simulink model "active_with_narx_and_can"  (R2024a)
settings: Solver=FixedStepAuto  StartTime=0.0  StopTime=40  FixedStep=0.005  RelTol=1e-3
undefined symbols (not defined in the file): A, B, C, canChannel, D, E, H, K1, K2, params, VehicleDataSingle
libraries: neural x41, j1939protocollib x5, vntj1939tllib x1, sldrtlib x1, simulink x1
(part 3 of 3)

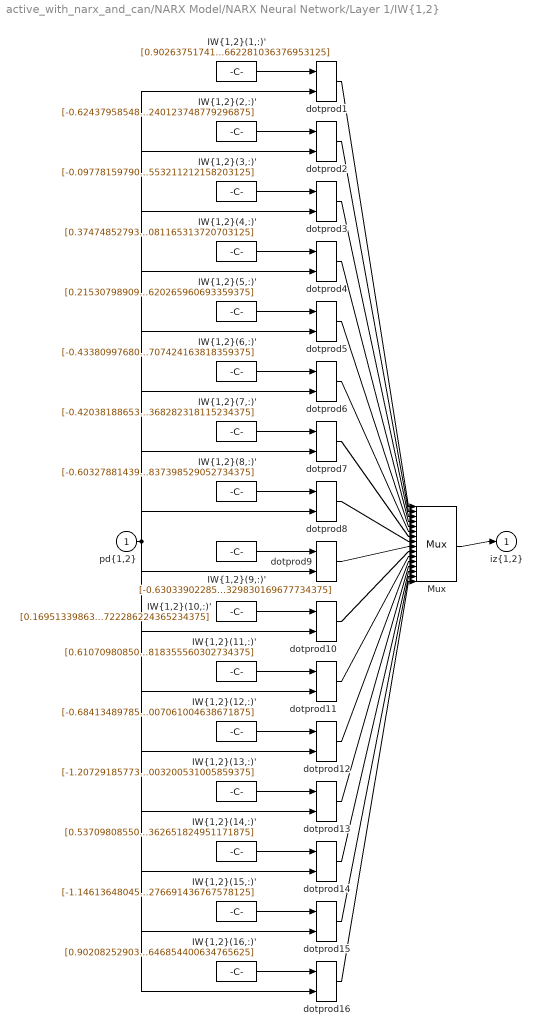
== system active_with_narx_and_can/NARX Model/NARX Neural Network/Layer 1/IW{1,2} ==
  "pd{1,2}" : Inport  PortDimensions=8
      mask Display: e = 0.06;c1 = [120 230 180]/255;c2 = ([120 230 180]+0)/(256+128);c3 = ([120 230 180]+128)/(256+128);patch([0 1 1 0],[0 0 1 1],c1);patch([0 1 1 1-e 1-e 0+e],[0 0 1 1-e 0+e 0+e],c2);patch([0 0 1 1-e 0+e 0+e],[0 1 1 1-e 1-e 0+e],c3);plot([0 1 1 0 0],[0 0 1 1 0]);
  "IW{1,2}(1,:)'" : Constant  Value=[0.90263751741286313290402176789939403533935546875;-0.21601499662720013983374656163505278527736663818359375;0.303445752325211037803143199198530055582523345947265625;-0.485376444032000919914793257703422568738460540771484375;0.23563832005407914227390619998914189636707305908203125;0.2294133098908705259422191602425300516188144683837890625;0.25051304698929321990163998634670861065387725830078125;0.1704435947606100232309955799792078323662281036376953125]
      mask Display: e = 0.06;c1 = [120 150 230]/255;c2 = ([120 150 230]+0)/383;c3 = ([120 150 230]+128)/383;patch([0 1 1 0],[0 0 1 1],c1);patch([0 1 1 1-e 1-e 0+e],[0 0 1 1-e 0+e 0+e],c2);patch([0 0 1 1-e 0+e 0+e],[0 1 1 1-e 1-e 0+e],c3);plot([0 1 1 0 0],[0 0 1 1 0]);disp('Weights');
  "IW{1,2}(10,:)'" : Constant  Value=[0.169513398630651845877537198248319327831268310546875;-1.0365359109949310312259740385343320667743682861328125;0.11236096590994171240396326538757421076297760009765625;-0.55860279468901430366400973070994950830936431884765625;0.40321310435647372827361323288641870021820068359375;0.2438622089058629927027510575499036349356174468994140625;0.218310799669648336607252758767572231590747833251953125;0.1471962379093022244003208243157132528722286224365234375]
      mask Display: e = 0.06;c1 = [120 150 230]/255;c2 = ([120 150 230]+0)/383;c3 = ([120 150 230]+128)/383;patch([0 1 1 0],[0 0 1 1],c1);patch([0 1 1 1-e 1-e 0+e],[0 0 1 1-e 0+e 0+e],c2);patch([0 0 1 1-e 0+e 0+e],[0 1 1 1-e 1-e 0+e],c3);plot([0 1 1 0 0],[0 0 1 1 0]);disp('Weights');
  "IW{1,2}(11,:)'" : Constant  Value=[0.61070980850982314880326384809450246393680572509765625;-0.6571629666322793550392589168041013181209564208984375;-0.292207907782760123449605771384085528552532196044921875;-0.6071086591404124543913667366723529994487762451171875;-0.7255795782161500451223901109187863767147064208984375;-0.10046686132956735015842042457734351046383380889892578125;-0.29501543782765649037713728830567561089992523193359375;-0.057419468308792909194693265817477367818355560302734375]
      mask Display: e = 0.06;c1 = [120 150 230]/255;c2 = ([120 150 230]+0)/383;c3 = ([120 150 230]+128)/383;patch([0 1 1 0],[0 0 1 1],c1);patch([0 1 1 1-e 1-e 0+e],[0 0 1 1-e 0+e 0+e],c2);patch([0 0 1 1-e 0+e 0+e],[0 1 1 1-e 1-e 0+e],c3);plot([0 1 1 0 0],[0 0 1 1 0]);disp('Weights');
  "IW{1,2}(12,:)'" : Constant  Value=[-0.68413489785069703241759953016298823058605194091796875;0.7251253878621028992057517825742252171039581298828125;-0.2162451686483140844696748672504327259957790374755859375;1.14689883587164676015390796237625181674957275390625;1.4145020007900115377452721077133901417255401611328125;-0.269077578797319028058865342245553620159626007080078125;0.00336010815578813813730985060601597069762647151947021484375;0.18742002039583638417497013506363146007061004638671875]
      mask Display: e = 0.06;c1 = [120 150 230]/255;c2 = ([120 150 230]+0)/383;c3 = ([120 150 230]+128)/383;patch([0 1 1 0],[0 0 1 1],c1);patch([0 1 1 1-e 1-e 0+e],[0 0 1 1-e 0+e 0+e],c2);patch([0 0 1 1-e 0+e 0+e],[0 1 1 1-e 1-e 0+e],c3);plot([0 1 1 0 0],[0 0 1 1 0]);disp('Weights');
  "IW{1,2}(13,:)'" : Constant  Value=[-1.207291857736213724905383060104213654994964599609375;-0.01499466201103569380770341723518868093378841876983642578125;-0.173091376080131309489473778739920817315578460693359375;0.282268142750107420280158976311213336884975433349609375;1.1083543211750790380420994551968760788440704345703125;-0.00180324813542519723184864854914621901116333901882171630859375;-0.4755764174158214618870488266111351549625396728515625;-0.696182258878252469003200531005859375]
      mask Display: e = 0.06;c1 = [120 150 230]/255;c2 = ([120 150 230]+0)/383;c3 = ([120 150 230]+128)/383;patch([0 1 1 0],[0 0 1 1],c1);patch([0 1 1 1-e 1-e 0+e],[0 0 1 1-e 0+e 0+e],c2);patch([0 0 1 1-e 0+e 0+e],[0 1 1 1-e 1-e 0+e],c3);plot([0 1 1 0 0],[0 0 1 1 0]);disp('Weights');
  "IW{1,2}(14,:)'" : Constant  Value=[0.5370980855067768455768373314640484750270843505859375;-0.313056847114534908538274748934782110154628753662109375;0.0770138039934813445341887927497737109661102294921875;0.64018782705027021950883181489189155399799346923828125;-0.07635916492874746108743266859164577908813953399658203125;0.0942864795317774895266893508960492908954620361328125;-0.09106729824357506775101001039729453623294830322265625;0.42317469894027837096217581347445957362651824951171875]
      mask Display: e = 0.06;c1 = [120 150 230]/255;c2 = ([120 150 230]+0)/383;c3 = ([120 150 230]+128)/383;patch([0 1 1 0],[0 0 1 1],c1);patch([0 1 1 1-e 1-e 0+e],[0 0 1 1-e 0+e 0+e],c2);patch([0 0 1 1-e 0+e 0+e],[0 1 1 1-e 1-e 0+e],c3);plot([0 1 1 0 0],[0 0 1 1 0]);disp('Weights');
  "IW{1,2}(15,:)'" : Constant  Value=[-1.146136480454412076568360134842805564403533935546875;-0.0944942787904399228438023783382959663867950439453125;-0.3428836995163557777033247475628741085529327392578125;-0.7923366916232279510978742109728045761585235595703125;-0.06468206728460264287594583265672554261982440948486328125;0.60584543936818746612260611072997562587261199951171875;0.768091475662020517489736448624171316623687744140625;0.63206824404375716586201860991423018276691436767578125]
      mask Display: e = 0.06;c1 = [120 150 230]/255;c2 = ([120 150 230]+0)/383;c3 = ([120 150 230]+128)/383;patch([0 1 1 0],[0 0 1 1],c1);patch([0 1 1 1-e 1-e 0+e],[0 0 1 1-e 0+e 0+e],c2);patch([0 0 1 1-e 0+e 0+e],[0 1 1 1-e 1-e 0+e],c3);plot([0 1 1 0 0],[0 0 1 1 0]);disp('Weights');
  "IW{1,2}(16,:)'" : Constant  Value=[0.90208252903466756844608198662172071635723114013671875;-0.36075579545011626780848246198729611933231353759765625;-0.47607267246013462713705166606814600527286529541015625;-0.4239340155265429732622806113795377314090728759765625;0.323166192061411561287087579330545850098133087158203125;-0.417318695834025199520311844025854952633380889892578125;-0.79057600537506467208714866501395590603351593017578125;-0.72856943152513642392165138517157174646854400634765625]
      mask Display: e = 0.06;c1 = [120 150 230]/255;c2 = ([120 150 230]+0)/383;c3 = ([120 150 230]+128)/383;patch([0 1 1 0],[0 0 1 1],c1);patch([0 1 1 1-e 1-e 0+e],[0 0 1 1-e 0+e 0+e],c2);patch([0 0 1 1-e 0+e 0+e],[0 1 1 1-e 1-e 0+e],c3);plot([0 1 1 0 0],[0 0 1 1 0]);disp('Weights');
  "IW{1,2}(2,:)'" : Constant  Value=[-0.62437958548816696602301590246497653424739837646484375;0.4030010330402535867477809006231836974620819091796875;-0.93345120950187820962895557386218570172786712646484375;-0.99941077496806574043120008354890160262584686279296875;-0.805871382932370039497982361353933811187744140625;-1.1641510599605722209304303760291077196598052978515625;-0.73810501632568803476175389732816256582736968994140625;-0.52273946016513750389975712096202187240123748779296875]
      mask Display: e = 0.06;c1 = [120 150 230]/255;c2 = ([120 150 230]+0)/383;c3 = ([120 150 230]+128)/383;patch([0 1 1 0],[0 0 1 1],c1);patch([0 1 1 1-e 1-e 0+e],[0 0 1 1-e 0+e 0+e],c2);patch([0 0 1 1-e 0+e 0+e],[0 1 1 1-e 1-e 0+e],c3);plot([0 1 1 0 0],[0 0 1 1 0]);disp('Weights');
  "IW{1,2}(3,:)'" : Constant  Value=[-0.09778159790864258960052524116690619848668575286865234375;-0.385707484802180811112037872590008191764354705810546875;0.7925023952755034795103483702405355870723724365234375;0.51074010904656663711875808076001703739166259765625;-0.68969065456008837866619387568789534270763397216796875;-0.00582392983700102083444161138459094217978417873382568359375;0.1302174028268628103166548726221662946045398712158203125;0.1331059726587587033197479513546568341553211212158203125]
      mask Display: e = 0.06;c1 = [120 150 230]/255;c2 = ([120 150 230]+0)/383;c3 = ([120 150 230]+128)/383;patch([0 1 1 0],[0 0 1 1],c1);patch([0 1 1 1-e 1-e 0+e],[0 0 1 1-e 0+e 0+e],c2);patch([0 0 1 1-e 0+e 0+e],[0 1 1 1-e 1-e 0+e],c3);plot([0 1 1 0 0],[0 0 1 1 0]);disp('Weights');
  "IW{1,2}(4,:)'" : Constant  Value=[0.37474852793019242103156329903868027031421661376953125;0.2591676118072852030849162474623881280422210693359375;-0.2053060696935578022248591878451406955718994140625;0.2190438597914983187564530453528277575969696044921875;-0.06545895398947572385583981713352841325104236602783203125;-0.2064269491545067669591162484721280634403228759765625;-0.11894725401665766362224729846275295130908489227294921875;0.0374038305425073158705373543853056617081165313720703125]
      mask Display: e = 0.06;c1 = [120 150 230]/255;c2 = ([120 150 230]+0)/383;c3 = ([120 150 230]+128)/383;patch([0 1 1 0],[0 0 1 1],c1);patch([0 1 1 1-e 1-e 0+e],[0 0 1 1-e 0+e 0+e],c2);patch([0 0 1 1-e 0+e 0+e],[0 1 1 1-e 1-e 0+e],c3);plot([0 1 1 0 0],[0 0 1 1 0]);disp('Weights');
  "IW{1,2}(5,:)'" : Constant  Value=[0.21530798909694393028502190645667724311351776123046875;-0.896805076954492630392223873059265315532684326171875;0.433263582933134439034716933747404254972934722900390625;-0.180462695486016289070363427526899613440036773681640625;0.32220381062158953699992025576648302376270294189453125;-0.1843317232416837592179348348508938215672969818115234375;0.35367194604087914822088123401044867932796478271484375;0.42561556904118302835371423498145304620265960693359375]
      mask Display: e = 0.06;c1 = [120 150 230]/255;c2 = ([120 150 230]+0)/383;c3 = ([120 150 230]+128)/383;patch([0 1 1 0],[0 0 1 1],c1);patch([0 1 1 1-e 1-e 0+e],[0 0 1 1-e 0+e 0+e],c2);patch([0 0 1 1-e 0+e 0+e],[0 1 1 1-e 1-e 0+e],c3);plot([0 1 1 0 0],[0 0 1 1 0]);disp('Weights');
  "IW{1,2}(6,:)'" : Constant  Value=[-0.433809976807434882761782546367612667381763458251953125;-0.270578592932165740148064969616825692355632781982421875;-0.4396279200653336882709254496148787438869476318359375;0.0907362057473349026270881267919321544468402862548828125;0.251838525357704512419587672411580570042133331298828125;-0.02289131637670037411336210197987384162843227386474609375;0.1623517875336642768413497606161399744451045989990234375;0.08045006984227652535590635807238868437707424163818359375]
      mask Display: e = 0.06;c1 = [120 150 230]/255;c2 = ([120 150 230]+0)/383;c3 = ([120 150 230]+128)/383;patch([0 1 1 0],[0 0 1 1],c1);patch([0 1 1 1-e 1-e 0+e],[0 0 1 1-e 0+e 0+e],c2);patch([0 0 1 1-e 0+e 0+e],[0 1 1 1-e 1-e 0+e],c3);plot([0 1 1 0 0],[0 0 1 1 0]);disp('Weights');
  "IW{1,2}(7,:)'" : Constant  Value=[-0.420381886532580295590122432258795015513896942138671875;0.18477735142202422746748879944789223372936248779296875;-0.48409542286411000322488007441279478371143341064453125;-0.2112447543197915333923475600386154837906360626220703125;-0.1131105735586611371612519860718748532235622406005859375;-0.268798366024736612445167338592000305652618408203125;-0.136020135754542526029808868770487606525421142578125;-0.0886993300823918084940800099502666853368282318115234375]
      mask Display: e = 0.06;c1 = [120 150 230]/255;c2 = ([120 150 230]+0)/383;c3 = ([120 150 230]+128)/383;patch([0 1 1 0],[0 0 1 1],c1);patch([0 1 1 1-e 1-e 0+e],[0 0 1 1-e 0+e 0+e],c2);patch([0 0 1 1-e 0+e 0+e],[0 1 1 1-e 1-e 0+e],c3);plot([0 1 1 0 0],[0 0 1 1 0]);disp('Weights');
  "IW{1,2}(8,:)'" : Constant  Value=[-0.603278814390159734415419734432362020015716552734375;0.1260379163613980224578625666254083625972270965576171875;0.227830739133030368837040668950066901743412017822265625;0.72188803288705416516535251503228209912776947021484375;0.942978873146900209434306816547177731990814208984375;0.9617318813040556246818368890671990811824798583984375;-0.386824720566464275162132935292902402579784393310546875;-0.0515663129788129503960902866310789249837398529052734375]
      mask Display: e = 0.06;c1 = [120 150 230]/255;c2 = ([120 150 230]+0)/383;c3 = ([120 150 230]+128)/383;patch([0 1 1 0],[0 0 1 1],c1);patch([0 1 1 1-e 1-e 0+e],[0 0 1 1-e 0+e 0+e],c2);patch([0 0 1 1-e 0+e 0+e],[0 1 1 1-e 1-e 0+e],c3);plot([0 1 1 0 0],[0 0 1 1 0]);disp('Weights');
  "IW{1,2}(9,:)'" : Constant  Value=[-0.63033902285547060984072231804020702838897705078125;-0.5593934237156599209583873744122684001922607421875;-0.413146987113548858072675784569582901895046234130859375;0.14086159676361831305513305778731591999530792236328125;-0.612650184316847035148612121702171862125396728515625;1.1652010827542447213289733554120175540447235107421875;-0.667181620491609894685325343743897974491119384765625;-0.51448630339249967757808690294041298329830169677734375]
      mask Display: e = 0.06;c1 = [120 150 230]/255;c2 = ([120 150 230]+0)/383;c3 = ([120 150 230]+128)/383;patch([0 1 1 0],[0 0 1 1],c1);patch([0 1 1 1-e 1-e 0+e],[0 0 1 1-e 0+e 0+e],c2);patch([0 0 1 1-e 0+e 0+e],[0 1 1 1-e 1-e 0+e],c3);plot([0 1 1 0 0],[0 0 1 1 0]);disp('Weights');
  Mux : Mux  Inputs=16
      mask Display: e = 0.06;c1 = [120 150 230]/255;c2 = ([120 150 230]+0)/383;c3 = ([120 150 230]+128)/383;patch([0 1 1 0],[0 0 1 1],c1);patch([0 1 1 1-e 1-e 0+e],[0 0 1 1-e 0+e 0+e],c2);patch([0 0 1 1-e 0+e 0+e],[0 1 1 1-e 1-e 0+e],c3);plot([0 1 1 0 0],[0 0 1 1 0]);disp('Mux');
  dotprod{1..16} (16 alike) : neural/Weight Functions/dotprod
  "iz{1,2}" : Outport
      mask Display: e = 0.06;c1 = [120 230 180]/255;c2 = ([120 230 180]+0)/(256+128);c3 = ([120 230 180]+128)/(256+128);patch([0 1 1 0],[0 0 1 1],c1);patch([0 1 1 1-e 1-e 0+e],[0 0 1 1-e 0+e 0+e],c2);patch([0 0 1 1-e 0+e 0+e],[0 1 1 1-e 1-e 0+e],c3);plot([0 1 1 0 0],[0 0 1 1 0]);
  wires:
  "IW{1,2}(1,:)'"/1 -> dotprod1/1
  "pd{1,2}"/1 -> dotprod1/2, dotprod2/2, dotprod3/2, dotprod4/2, dotprod5/2, dotprod6/2, dotprod7/2, dotprod8/2, dotprod9/2, dotprod10/2, dotprod11/2, dotprod12/2, dotprod13/2, dotprod14/2, dotprod15/2, dotprod16/2
  dotprod1/1 -> Mux/1
  "IW{1,2}(2,:)'"/1 -> dotprod2/1
  dotprod2/1 -> Mux/2
  "IW{1,2}(3,:)'"/1 -> dotprod3/1
  dotprod3/1 -> Mux/3
  "IW{1,2}(4,:)'"/1 -> dotprod4/1
  dotprod4/1 -> Mux/4
  "IW{1,2}(5,:)'"/1 -> dotprod5/1
  dotprod5/1 -> Mux/5
  "IW{1,2}(6,:)'"/1 -> dotprod6/1
  dotprod6/1 -> Mux/6
  "IW{1,2}(7,:)'"/1 -> dotprod7/1
  dotprod7/1 -> Mux/7
  "IW{1,2}(8,:)'"/1 -> dotprod8/1
  dotprod8/1 -> Mux/8
  "IW{1,2}(9,:)'"/1 -> dotprod9/1
  dotprod9/1 -> Mux/9
  "IW{1,2}(10,:)'"/1 -> dotprod10/1
  dotprod10/1 -> Mux/10
  "IW{1,2}(11,:)'"/1 -> dotprod11/1
  dotprod11/1 -> Mux/11
  "IW{1,2}(12,:)'"/1 -> dotprod12/1
  dotprod12/1 -> Mux/12
  "IW{1,2}(13,:)'"/1 -> dotprod13/1
  dotprod13/1 -> Mux/13
  "IW{1,2}(14,:)'"/1 -> dotprod14/1
  dotprod14/1 -> Mux/14
  "IW{1,2}(15,:)'"/1 -> dotprod15/1
  dotprod15/1 -> Mux/15
  "IW{1,2}(16,:)'"/1 -> dotprod16/1
  dotprod16/1 -> Mux/16
  Mux/1 -> "iz{1,2}"/1

== system active_with_narx_and_can/NARX Model/NARX Neural Network/Layer 2/Delays 1 ==
  "p{2}" : Inport  PortDimensions=16
      mask Display: e = 0.06;c1 = [120 230 180]/255;c2 = ([120 230 180]+0)/(256+128);c3 = ([120 230 180]+128)/(256+128);patch([0 1 1 0],[0 0 1 1],c1);patch([0 1 1 1-e 1-e 0+e],[0 0 1 1-e 0+e 0+e],c2);patch([0 0 1 1-e 0+e 0+e],[0 1 1 1-e 1-e 0+e],c3);plot([0 1 1 0 0],[0 0 1 1 0]);
  mux : Mux  Inputs=1
      mask Display: e = 0.06;c1 = [120 150 230]/255;c2 = ([120 150 230]+0)/383;c3 = ([120 150 230]+128)/383;patch([0 1 1 0],[0 0 1 1],c1);patch([0 1 1 1-e 1-e 0+e],[0 0 1 1-e 0+e 0+e],c2);patch([0 0 1 1-e 0+e 0+e],[0 1 1 1-e 1-e 0+e],c3);plot([0 1 1 0 0],[0 0 1 1 0]);disp('Mux')
  "pd{2,1}" : Outport
      mask Display: e = 0.06;c1 = [120 230 180]/255;c2 = ([120 230 180]+0)/(256+128);c3 = ([120 230 180]+128)/(256+128);patch([0 1 1 0],[0 0 1 1],c1);patch([0 1 1 1-e 1-e 0+e],[0 0 1 1-e 0+e 0+e],c2);patch([0 0 1 1-e 0+e 0+e],[0 1 1 1-e 1-e 0+e],c3);plot([0 1 1 0 0],[0 0 1 1 0]);
  wires:
  "p{2}"/1 -> mux/1
  mux/1 -> "pd{2,1}"/1

== system active_with_narx_and_can/NARX Model/NARX Neural Network/Layer 2/LW{2,1} ==
  "ad{2,1}" : Inport  PortDimensions=16
      mask Display: e = 0.06;c1 = [120 230 180]/255;c2 = ([120 230 180]+0)/(256+128);c3 = ([120 230 180]+128)/(256+128);patch([0 1 1 0],[0 0 1 1],c1);patch([0 1 1 1-e 1-e 0+e],[0 0 1 1-e 0+e 0+e],c2);patch([0 0 1 1-e 0+e 0+e],[0 1 1 1-e 1-e 0+e],c3);plot([0 1 1 0 0],[0 0 1 1 0]);
  "IW{2,1}(1,:)'" : Constant  Value=[-0.037283359326283883883323966301759355701506137847900390625;-0.00752528952071175420701631963993349927477538585662841796875;-0.064064462501762398094484751709387637674808502197265625;1.062458244357101566635037670494057238101959228515625;0.035078437349624867758191015809643431566655635833740234375;-0.0231289547996484136371808659760063164867460727691650390625;-0.86705623148364552310596309325774200260639190673828125;-0.1254112477086657129188296266875113360583782196044921875;0.041761451141637866146805180278533953242003917694091796875;-0.159013841309073866714385303566814400255680084228515625;0.15100937644207623744563306900090537965297698974609375;-0.08639823493543609400635574502302915789186954498291015625;0.381990846404795636459539309726096689701080322265625;0.041620895665299674492931814029361703433096408843994140625;0.69392710050268091581671114909113384783267974853515625;0.32302310650360721577811773386201821267604827880859375]
      mask Display: e = 0.06;c1 = [120 150 230]/255;c2 = ([120 150 230]+0)/383;c3 = ([120 150 230]+128)/383;patch([0 1 1 0],[0 0 1 1],c1);patch([0 1 1 1-e 1-e 0+e],[0 0 1 1-e 0+e 0+e],c2);patch([0 0 1 1-e 0+e 0+e],[0 1 1 1-e 1-e 0+e],c3);plot([0 1 1 0 0],[0 0 1 1 0]);disp('weights');
  "IW{2,1}(2,:)'" : Constant  Value=[0.5111938979159684759423498690011911094188690185546875;0.56569826864207206629231450278894044458866119384765625;-0.2022808398030029319869527171249501407146453857421875;0.43664179142422965274050739026279188692569732666015625;-0.023148512601576298752803495517582632601261138916015625;-0.039420645504728957231321828658110462129116058349609375;-0.443177042395416720399481391723384149372577667236328125;0.1251048868280779657879975275136530399322509765625;0.315708570588528580902476505798404105007648468017578125;0.10083913826751049469532262037319014780223369598388671875;-1.014326253145053424731258928659372031688690185546875;-0.154106037329089229359624368953518569469451904296875;-0.181478084800968275658306083641946315765380859375;-0.4660474982754012618357819519587792456150054931640625;-0.047110076733224336142935584348379052244126796722412109375;-0.01314367972709637628903056594253939692862331867218017578125]
      mask Display: e = 0.06;c1 = [120 150 230]/255;c2 = ([120 150 230]+0)/383;c3 = ([120 150 230]+128)/383;patch([0 1 1 0],[0 0 1 1],c1);patch([0 1 1 1-e 1-e 0+e],[0 0 1 1-e 0+e 0+e],c2);patch([0 0 1 1-e 0+e 0+e],[0 1 1 1-e 1-e 0+e],c3);plot([0 1 1 0 0],[0 0 1 1 0]);disp('weights');
  "IW{2,1}(3,:)'" : Constant  Value=[1.933346201116522333762759444653056561946868896484375;1.0965223692714347603072155834524892270565032958984375;2.11297243584186045239903251058422029018402099609375;0.52748544965964405673020110043580643832683563232421875;-1.0002554175522553325805574786500073969364166259765625;0.8390816199270270114851655307575128972530364990234375;0.48619722837803969195391573521192185580730438232421875;1.74443508109092082491997643955983221530914306640625;0.6463893650373344623716320711537264287471771240234375;1.328196156840519837061265207012183964252471923828125;1.2321513257421383702450157215935178101062774658203125;1.89817934085664941079585332772694528102874755859375;-1.56555390572099373258652121876366436481475830078125;-2.02506016769746199912560769007541239261627197265625;-2.046024633954304672300850143074057996273040771484375;-0.8677617795247083432030876792850904166698455810546875]
      mask Display: e = 0.06;c1 = [120 150 230]/255;c2 = ([120 150 230]+0)/383;c3 = ([120 150 230]+128)/383;patch([0 1 1 0],[0 0 1 1],c1);patch([0 1 1 1-e 1-e 0+e],[0 0 1 1-e 0+e 0+e],c2);patch([0 0 1 1-e 0+e 0+e],[0 1 1 1-e 1-e 0+e],c3);plot([0 1 1 0 0],[0 0 1 1 0]);disp('weights');
  "IW{2,1}(4,:)'" : Constant  Value=[-1.7417245186385326150002583744935691356658935546875;-0.957382664117269133186027829651720821857452392578125;-1.8871798005697486555476416469900868833065032958984375;-0.91295989683833822514458233854384161531925201416015625;0.91955159516746942660603281183284707367420196533203125;-0.746688674045671962886672190506942570209503173828125;-1.1816807626701673061830888400436379015445709228515625;-1.5862227610216377282625899169943295419216156005859375;-0.69865648831194648860076767959981225430965423583984375;-1.3350977810611708296306687770993448793888092041015625;-1.022288805661370592048342587077058851718902587890625;-1.597547998778193534263891706359572708606719970703125;1.159446134005739370564924684003926813602447509765625;1.78006360541741148750816137180663645267486572265625;1.3244675034032111771153950030566193163394927978515625;0.5186953652995283103877000030479393899440765380859375]
      mask Display: e = 0.06;c1 = [120 150 230]/255;c2 = ([120 150 230]+0)/383;c3 = ([120 150 230]+128)/383;patch([0 1 1 0],[0 0 1 1],c1);patch([0 1 1 1-e 1-e 0+e],[0 0 1 1-e 0+e 0+e],c2);patch([0 0 1 1-e 0+e 0+e],[0 1 1 1-e 1-e 0+e],c3);plot([0 1 1 0 0],[0 0 1 1 0]);disp('weights');
  Mux : Mux
      mask Display: e = 0.06;c1 = [120 150 230]/255;c2 = ([120 150 230]+0)/383;c3 = ([120 150 230]+128)/383;patch([0 1 1 0],[0 0 1 1],c1);patch([0 1 1 1-e 1-e 0+e],[0 0 1 1-e 0+e 0+e],c2);patch([0 0 1 1-e 0+e 0+e],[0 1 1 1-e 1-e 0+e],c3);plot([0 1 1 0 0],[0 0 1 1 0]);disp('Mux');
  dotprod{1..4} (4 alike) : neural/Weight Functions/dotprod
  "lz{2,1}" : Outport
      mask Display: e = 0.06;c1 = [120 230 180]/255;c2 = ([120 230 180]+0)/(256+128);c3 = ([120 230 180]+128)/(256+128);patch([0 1 1 0],[0 0 1 1],c1);patch([0 1 1 1-e 1-e 0+e],[0 0 1 1-e 0+e 0+e],c2);patch([0 0 1 1-e 0+e 0+e],[0 1 1 1-e 1-e 0+e],c3);plot([0 1 1 0 0],[0 0 1 1 0]);
  wires:
  "IW{2,1}(1,:)'"/1 -> dotprod1/1
  "ad{2,1}"/1 -> dotprod1/2, dotprod2/2, dotprod3/2, dotprod4/2
  dotprod1/1 -> Mux/1
  "IW{2,1}(2,:)'"/1 -> dotprod2/1
  dotprod2/1 -> Mux/2
  "IW{2,1}(3,:)'"/1 -> dotprod3/1
  dotprod3/1 -> Mux/3
  "IW{2,1}(4,:)'"/1 -> dotprod4/1
  dotprod4/1 -> Mux/4
  Mux/1 -> "lz{2,1}"/1

== matlab function active_with_narx_and_can/Motor Model/force/MATLAB Function2 ==
  data: y input; F output; u input; F3max input; F3min input; F4max input; F4min input
function F = fcn(y, u, F3max, F3min, F4max, F4min)
if y == 1
    F = u;
elseif y == 2
    F = u;
elseif y == 3
    if u > F3max
        F = F3max;
    elseif u < F3min
        F = F3min;
    else
        F = u;
    end
else
    % elseif y==4
    if u > F4max
        F = F4max;
    elseif u < F4min
        F = F4min;
    else
        F = u;
    end
end

== matlab function active_with_narx_and_can/Motor Model/force/MATLAB Function6 ==
  data: y input; F output; u input; F3max input; F3min input; F4max input; F4min input
function F = fcn(y, u, F3max, F3min, F4max, F4min)
if y == 1
    F = u;
elseif y == 2
    F = u;
elseif y == 3
    if u > F3max
        F = F3max;
    elseif u < F3min
        F = F3min;
    else
        F = u;
    end
else
    % elseif y==4
    if u > F4max
        F = F4max;
    elseif u < F4min
        F = F4min;
    else
        F = u;
    end
end

== matlab function active_with_narx_and_can/NARX Data/MATLAB Function ==
  data: dX input; dx8 output; dx14 output
function [dx8, dx14] = fcn(dX)
dx8 = dX(8);
dx14 = dX(14);

== matlab function active_with_narx_and_can/NARX Model/MATLAB Function1 ==
  data: X input; x2 output; x4 output; x6 output; x7 output; x8 output; x13 output; x14 output
function [x2, x4, x6, x7, x8, x13, x14] = fcn(X)
x2 = X(2);
x4 = X(4);
x6 = X(6);
x7 = X(7);
x8 = X(8);
x13 = X(13);
x14 = X(14);

== matlab function active_with_narx_and_can/Motor Model/force/MATLAB Function1 ==
  data: y input; F output; u input; F3max input; F3min input; F4max input; F4min input
function F = fcn(y, u, F3max, F3min, F4max, F4min)
if y == 1
    F = u;
elseif y == 2
    F = u;
elseif y == 3
    if u > F3max
        F = F3max;
    elseif u < F3min
        F = F3min;
    else
        F = u;
    end
else
    % elseif y==4
    if u > F4max
        F = F4max;
    elseif u < F4min
        F = F4min;
    else
        F = u;
    end
end

== matlab function active_with_narx_and_can/NARX Model/MATLAB Function2 ==
  data: Y input; y4 output; y7 output
function [y4, y7] = fcn(Y)
y4 = Y(4);
y7 = Y(7);

== matlab function active_with_narx_and_can/LQR Controller/MATLAB Function2 ==
  data: w input; qt1 output; qt2 output; qt3 output; qt4 output
function [qt1, qt2, qt3, qt4] = fcn(w)
qt1 = w(1);
qt2 = w(2);
qt3 = w(3);
qt4 = w(4);

== matlab function active_with_narx_and_can/J1939 Transmition/ Periodic Trigger/Timer/MATLAB Function ==
  data: y output double
function y = fcn
%#codegen
persistent temp;
coder.extrinsic('tic')
if isempty(temp)
    tic;
    temp = 0;
end
coder.extrinsic('toc')
temp = toc;
y = temp;

== matlab function active_with_narx_and_can/J1939 Transmition/MATLAB Function1 ==
  data: u1 input; U output; u2 input; u3 input; u4 input
function U = fcn(u1, u2, u3, u4)

U = [u1, u2, u3, u4];

end

== matlab function active_with_narx_and_can/J1939 Transmition/MATLAB Function2 ==
  data: U input; u1 output; u2 output; u3 output; u4 output
function [u1, u2, u3, u4] = fcn(U)
u1 = U(1);
u2 = U(2);
u3 = U(3);
u4 = U(4);

== matlab function active_with_narx_and_can/Motor Model/MATLAB Function1 ==
  data: X input; x2 output; x4 output; x6 output; x8 output; x10 output; x12 output; x14 output
function [x2, x4, x6, x8, x10, x12, x14] = fcn(X)
x2 = X(2);
x4 = X(4);
x6 = X(6);
x8 = X(8);
x10 = X(10);
x12 = X(12);
x14 = X(14);

== matlab function active_with_narx_and_can/Motor Model/MATLAB Function ==
  data: U input; u1 output; u2 output; u3 output; u4 output
function [u1, u2, u3, u4] = fcn(U)
u1 = U(1);
u2 = U(2);
u3 = U(3);
u4 = U(4);

== matlab function active_with_narx_and_can/Motor Model/mode/MATLAB Function1 ==
  data: v input; u input; y output; u_min input; E input; U0 input
function y = fcn(v, u, u_min, E, U0)
if v * u >= 0
    y = 1;
elseif v * u < 0 && u > u_min
    y = 2;
elseif v * u < 0 && u <= u_min && E > U0
    y = 3;
else
    % elseif v*u<0 && u<=u_min && E<=U0
    y = 4;
end

== matlab function active_with_narx_and_can/Motor Model/mode/MATLAB Function2 ==
  data: v input; u input; y output; u_min input; E input; U0 input
function y = fcn(v, u, u_min, E, U0)
if v * u >= 0
    y = 1;
elseif v * u < 0 && u > u_min
    y = 2;
elseif v * u < 0 && u <= u_min && E > U0
    y = 3;
else
    % elseif v*u<0 && u<=u_min && E<=U0
    y = 4;
end

== matlab function active_with_narx_and_can/Motor Model/force/MATLAB Function5 ==
  data: y input; F output; u input; F3max input; F3min input; F4max input; F4min input
function F = fcn(y, u, F3max, F3min, F4max, F4min)
if y == 1
    F = u;
elseif y == 2
    F = u;
elseif y == 3
    if u > F3max
        F = F3max;
    elseif u < F3min
        F = F3min;
    else
        F = u;
    end
else
    % elseif y==4
    if u > F4max
        F = F4max;
    elseif u < F4min
        F = F4min;
    else
        F = u;
    end
end

== matlab function active_with_narx_and_can/Motor Model/mode/MATLAB Function4 ==
  data: v input; u input; y output; u_min input; E input; U0 input
function y = fcn(v, u, u_min, E, U0)
if v * u >= 0
    y = 1;
elseif v * u < 0 && u > u_min
    y = 2;
elseif v * u < 0 && u <= u_min && E > U0
    y = 3;
else
    % elseif v*u<0 && u<=u_min && E<=U0
    y = 4;
end

== matlab function active_with_narx_and_can/Motor Model/mode/MATLAB Function ==
  data: v input; u input; y output; u_min input; E input; U0 input
function y = fcn(v, u, u_min, E, U0)
if v * u >= 0
    y = 1;
elseif v * u < 0 && u > u_min
    y = 2;
elseif v * u < 0 && u <= u_min && E > U0
    y = 3;
else
    % elseif v*u<0 && u<=u_min && E<=U0
    y = 4;
end
